simulink model "IBSMC_f"  (R2016b)
settings: Solver=VariableStepAuto  StartTime=0.0  StopTime=0.1  RelTol=1e-3
values from neighbouring files (symbols this model uses):
  a1 = 0.5*eye(3)    [cons2.m]
  a2 = 0.5*eye(3)    [cons2.m]
  j = diag([2.35e-3 2.35e-3 5.26e-2])    [cons2.m]
  k1 = 0.5*eye(3)    [cons2.m]
  k2 = 10*eye(3)    [cons2.m]
undefined symbols (not defined in the file or in its folder): q1, q2
libraries: aerolibutil x1
settings Model: Creator=Ali  LastModifiedBy=Ali

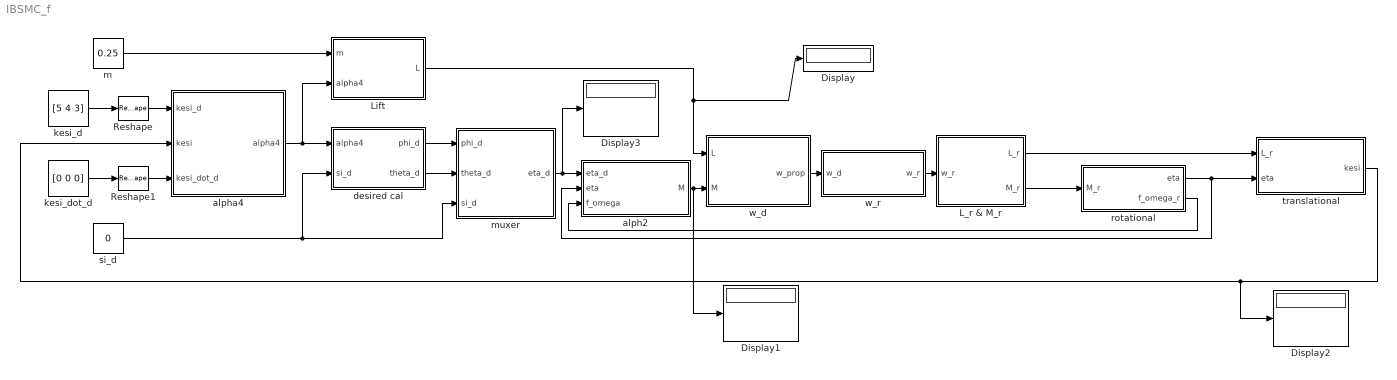
== system IBSMC_f ==
  Display{,1..3} (4 alike) : Display
  L_r & M_r : MATLAB Function  TreatAsAtomicUnit=on
  Lift : MATLAB Function  TreatAsAtomicUnit=on
  Reshape : Reshape  OutputDimensionality=Column vector (2-D)
  Reshape1 : Reshape  OutputDimensionality=Column vector (2-D)
  alph2 : Subsystem
  alpha4 : Subsystem
  desired cal : MATLAB Function  TreatAsAtomicUnit=on
  kesi_d : Constant  Value=[5 4 3]
  kesi_dot_d : Constant  Value=[0 0 0]
  m : Constant  Value=0.25
  muxer : MATLAB Function  TreatAsAtomicUnit=on
  rotational : Subsystem
  si_d : Constant  Value=0
  translational : Subsystem
  w_d : MATLAB Function  TreatAsAtomicUnit=on
  w_r : Subsystem
  wires:
  si_d/1 -> muxer/3(si_d), desired cal/2(si_d)
  desired cal/1(phi_d) -> muxer/1(phi_d)
  desired cal/2(theta_d) -> muxer/2(theta_d)
  muxer/1(eta_d) -> Display3/1, alph2/1(eta_d)
  alpha4/1(alpha4) -> desired cal/1(alpha4), Lift/2(alpha4)
  m/1 -> Lift/1(m)
  alph2/1(M) -> Display1/1, w_d/2(M)
  Lift/1(L) -> Display/1, w_d/1(L)
  w_d/1(w_prop) -> w_r/1(w_d)
  w_r/1(w_r) -> L_r & M_r/1(w_r)
  L_r & M_r/2(M_r) -> rotational/1(M_r)
  rotational/2(f_omega_r) -> alph2/3(f_omega)
  rotational/1(eta) -> alph2/2(eta), translational/2(eta)
  L_r & M_r/1(L_r) -> translational/1(L_r)
  translational/1(kesi) -> alpha4/2(kesi), Display2/1
  Reshape/1 -> alpha4/1(kesi_d)
  kesi_d/1 -> Reshape/1
  Reshape1/1 -> alpha4/3(kesi_dot_d)
  kesi_dot_d/1 -> Reshape1/1

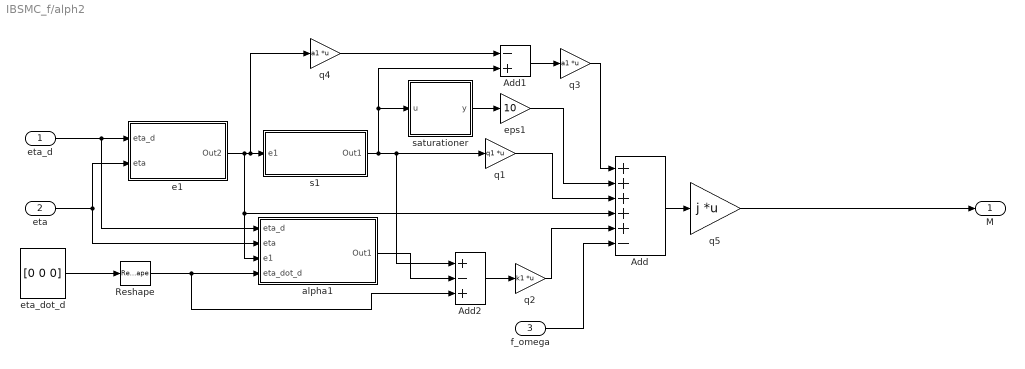
== system IBSMC_f/alph2 ==
  eta_d : Inport
  eta : Inport  Port=2
  f_omega : Inport  Port=3
  Add : Sum  Inputs=+++++-
  Add1 : Sum  Inputs=-+
  Add2 : Sum  Inputs=+-+
  Reshape : Reshape  OutputDimensionality=Column vector (2-D)
  alpha1 : Subsystem
  e1 : Subsystem
  eps1 : Gain  Gain=10
  eta_dot_d : Constant  Value=[0 0 0]
  q1 : Gain  Gain=q1  Multiplication=Matrix(K*u)
  q2 : Gain  Gain=k1  Multiplication=Matrix(K*u)
  q3 : Gain  Gain=a1  Multiplication=Matrix(K*u)
  q4 : Gain  Gain=a1  Multiplication=Matrix(K*u)
  q5 : Gain  Gain=j  Multiplication=Matrix(K*u)
  s1 : Subsystem
  saturationer : MATLAB Function  TreatAsAtomicUnit=on
  M : Outport
  wires:
  eta_d/1 -> alpha1/1(eta_d), e1/1(eta_d)
  e1/1(Out2) -> q4/1, s1/1(e1), alpha1/3(e1), Add/4
  eta_dot_d/1 -> Reshape/1
  saturationer/1(y) -> eps1/1
  s1/1(Out1) -> q1/1, Add2/1, saturationer/1(u), Add1/2
  q5/1 -> M/1
  q1/1 -> Add/3
  eps1/1 -> Add/2
  f_omega/1 -> Add/6
  alpha1/1(Out1) -> Add2/2
  Add2/1 -> q2/1
  q2/1 -> Add/5
  q3/1 -> Add/1
  Add1/1 -> q3/1
  q4/1 -> Add1/1
  eta/1 -> e1/2(eta), alpha1/2(eta)
  Add/1 -> q5/1
  Reshape/1 -> Add2/3, alpha1/4(eta_dot_d)

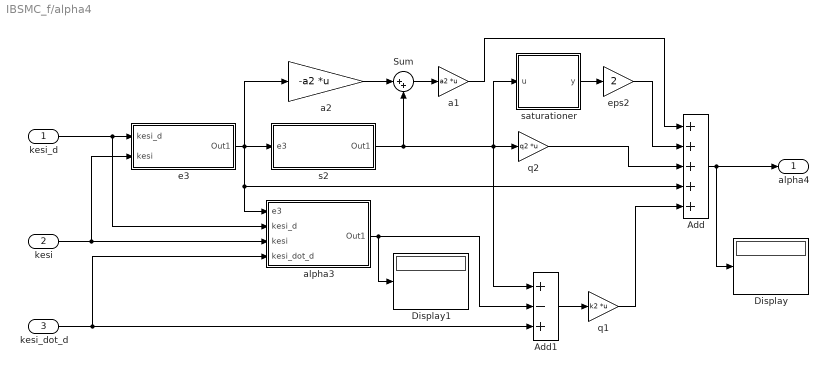
== system IBSMC_f/alpha4 ==
  kesi_d : Inport
  kesi : Inport  Port=2
  kesi_dot_d : Inport  Port=3
  Add : Sum  Inputs=+++++
  Add1 : Sum  Inputs=+-+
  Display : Display
  Display1 : Display
  Sum : Sum  Inputs=|++
  a1 : Gain  Gain=a2  Multiplication=Matrix(K*u)
  a2 : Gain  Gain=-a2  Multiplication=Matrix(K*u)
  alpha3 : Subsystem
  e3 : Subsystem
  eps2 : Gain  Gain=2
  q1 : Gain  Gain=k2  Multiplication=Matrix(K*u)
  q2 : Gain  Gain=q2  Multiplication=Matrix(K*u)
  s2 : Subsystem
  saturationer : MATLAB Function  TreatAsAtomicUnit=on
  alpha4 : Outport
  wires:
  saturationer/1(y) -> eps2/1
  q2/1 -> Add/3
  alpha3/1(Out1) -> Add1/2, Display1/1
  kesi/1 -> e3/2(kesi), alpha3/3(kesi)
  s2/1(Out1) -> q2/1, saturationer/1(u), Add1/1, Sum/2
  e3/1(Out1) -> s2/1(e3), alpha3/1(e3), Add/4, a2/1
  kesi_dot_d/1 -> alpha3/4(kesi_dot_d), Add1/3
  kesi_d/1 -> e3/1(kesi_d), alpha3/2(kesi_d)
  a2/1 -> Sum/1
  Sum/1 -> a1/1
  Add/1 -> alpha4/1, Display/1
  a1/1 -> Add/1
  Add1/1 -> q1/1
  q1/1 -> Add/5
  eps2/1 -> Add/2

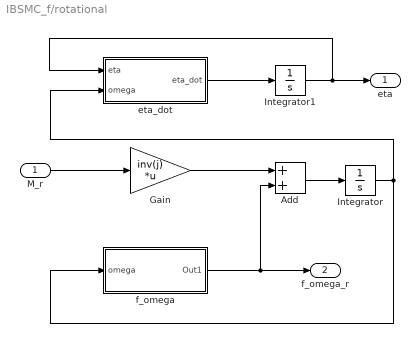
== system IBSMC_f/rotational ==
  M_r : Inport
  Add : Sum
  Gain : Gain  Gain=inv(j)  Multiplication=Matrix(K*u)
  Integrator : Integrator
  Integrator1 : Integrator
  eta_dot : Subsystem
  f_omega : Subsystem
  eta : Outport
  f_omega_r : Outport  Port=2
  wires:
  M_r/1 -> Gain/1
  Gain/1 -> Add/1
  Add/1 -> Integrator/1
  f_omega/1(Out1) -> Add/2, f_omega_r/1
  Integrator/1 -> f_omega/1(omega), eta_dot/2(omega)
  eta_dot/1(eta_dot) -> Integrator1/1
  Integrator1/1 -> eta/1, eta_dot/1(eta)

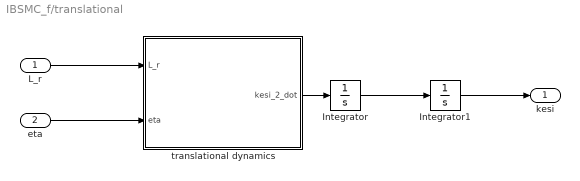
== system IBSMC_f/translational ==
  L_r : Inport
  eta : Inport  Port=2
  Integrator : Integrator
  Integrator1 : Integrator
  translational dynamics : MATLAB Function  TreatAsAtomicUnit=on
  kesi : Outport
  wires:
  L_r/1 -> translational dynamics/1(L_r)
  eta/1 -> translational dynamics/2(eta)
  Integrator/1 -> Integrator1/1
  translational dynamics/1(kesi_2_dot) -> Integrator/1
  Integrator1/1 -> kesi/1

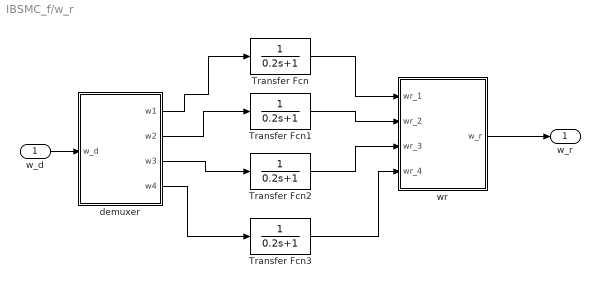
== system IBSMC_f/w_r ==
  w_d : Inport
  Transfer Fcn{,1..3} (4 alike) : TransferFcn  Denominator=[0.2 1]
  demuxer : MATLAB Function  TreatAsAtomicUnit=on
  wr : MATLAB Function  TreatAsAtomicUnit=on
  w_r : Outport
  wires:
  w_d/1 -> demuxer/1(w_d)
  demuxer/1(w1) -> Transfer Fcn/1
  demuxer/2(w2) -> Transfer Fcn1/1
  demuxer/3(w3) -> Transfer Fcn2/1
  demuxer/4(w4) -> Transfer Fcn3/1
  Transfer Fcn/1 -> wr/1(wr_1)
  Transfer Fcn1/1 -> wr/2(wr_2)
  Transfer Fcn2/1 -> wr/3(wr_3)
  Transfer Fcn3/1 -> wr/4(wr_4)
  wr/1(w_r) -> w_r/1

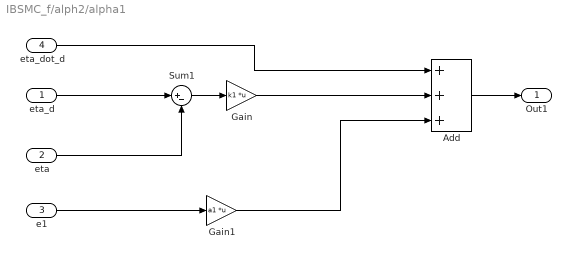
== system IBSMC_f/alph2/alpha1 ==
  eta_d : Inport
  eta : Inport  Port=2
  e1 : Inport  Port=3
  eta_dot_d : Inport  Port=4
  Add : Sum  Inputs=+++
  Gain : Gain  Gain=k1  Multiplication=Matrix(K*u)
  Gain1 : Gain  Gain=a1  Multiplication=Matrix(K*u)
  Sum1 : Sum  Inputs=|+-
  Out1 : Outport
  wires:
  Add/1 -> Out1/1
  Sum1/1 -> Gain/1
  eta/1 -> Sum1/2
  eta_d/1 -> Sum1/1
  Gain/1 -> Add/2
  eta_dot_d/1 -> Add/1
  e1/1 -> Gain1/1
  Gain1/1 -> Add/3

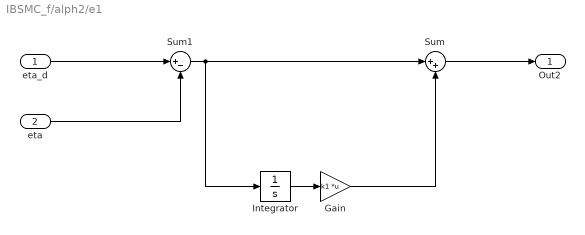
== system IBSMC_f/alph2/e1 ==
  eta_d : Inport
  eta : Inport  Port=2
  Gain : Gain  Gain=k1  Multiplication=Matrix(K*u)
  Integrator : Integrator
  Sum : Sum  Inputs=|++
  Sum1 : Sum  Inputs=|+-
  Out2 : Outport
  wires:
  eta_d/1 -> Sum1/1
  eta/1 -> Sum1/2
  Sum1/1 -> Integrator/1, Sum/1
  Sum/1 -> Out2/1
  Gain/1 -> Sum/2
  Integrator/1 -> Gain/1

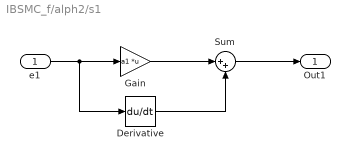
== system IBSMC_f/alph2/s1 ==
  e1 : Inport
  Derivative : Derivative
  Gain : Gain  Gain=a1  Multiplication=Matrix(K*u)
  Sum : Sum  Inputs=|++
  Out1 : Outport
  wires:
  Sum/1 -> Out1/1
  e1/1 -> Derivative/1, Gain/1
  Gain/1 -> Sum/1
  Derivative/1 -> Sum/2

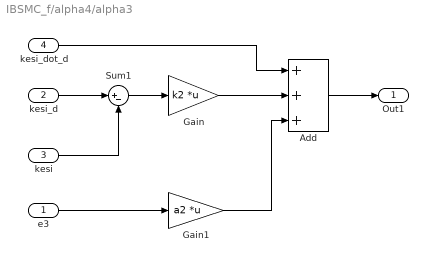
== system IBSMC_f/alpha4/alpha3 ==
  e3 : Inport
  kesi_d : Inport  Port=2
  kesi : Inport  Port=3
  kesi_dot_d : Inport  Port=4
  Add : Sum  Inputs=+++
  Gain : Gain  Gain=k2  Multiplication=Matrix(K*u)
  Gain1 : Gain  Gain=a2  Multiplication=Matrix(K*u)
  Sum1 : Sum  Inputs=|+-
  Out1 : Outport
  wires:
  Add/1 -> Out1/1
  Sum1/1 -> Gain/1
  kesi/1 -> Sum1/2
  kesi_d/1 -> Sum1/1
  Gain/1 -> Add/2
  kesi_dot_d/1 -> Add/1
  e3/1 -> Gain1/1
  Gain1/1 -> Add/3

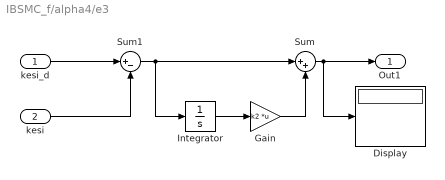
== system IBSMC_f/alpha4/e3 ==
  kesi_d : Inport
  kesi : Inport  Port=2
  Display : Display
  Gain : Gain  Gain=k2  Multiplication=Matrix(K*u)
  Integrator : Integrator
  Sum : Sum  Inputs=|++
  Sum1 : Sum  Inputs=|+-
  Out1 : Outport
  wires:
  kesi_d/1 -> Sum1/1
  kesi/1 -> Sum1/2
  Sum1/1 -> Integrator/1, Sum/1
  Integrator/1 -> Gain/1
  Gain/1 -> Sum/2
  Sum/1 -> Out1/1, Display/1

== system IBSMC_f/alpha4/s2 ==
  e3 : Inport
  Derivative : Derivative
  Gain : Gain  Gain=a2  Multiplication=Matrix(K*u)
  Sum : Sum  Inputs=|++
  Out1 : Outport
  wires:
  Sum/1 -> Out1/1
  e3/1 -> Derivative/1, Gain/1
  Gain/1 -> Sum/1
  Derivative/1 -> Sum/2

== system IBSMC_f/rotational/eta_dot ==
  eta : Inport
  omega : Inport  Port=2
  eta_dot_cal : MATLAB Function  TreatAsAtomicUnit=on
  eta_dot : Outport
  wires:
  eta_dot_cal/1(eta_dot) -> eta_dot/1
  eta/1 -> eta_dot_cal/1(eta)
  omega/1 -> eta_dot_cal/2(omega)

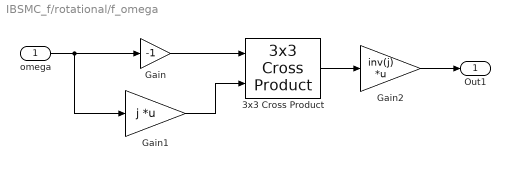
== system IBSMC_f/rotational/f_omega ==
  omega : Inport
  3x3 Cross Product : aerolibutil/3x3 Cross Product
  Gain : Gain  Gain=-1
  Gain1 : Gain  Gain=j  Multiplication=Matrix(K*u)
  Gain2 : Gain  Gain=inv(j)  Multiplication=Matrix(K*u)
  Out1 : Outport
  wires:
  omega/1 -> Gain1/1, Gain/1
  Gain/1 -> 3x3 Cross Product/1
  Gain1/1 -> 3x3 Cross Product/2
  3x3 Cross Product/1 -> Gain2/1
  Gain2/1 -> Out1/1

== matlab function IBSMC_f/desired cal ==
  data: alpha4 input; phi_d output; theta_d output; si_d input
function [phi_d,theta_d] = fcn(alpha4,si_d)
g=9.81;
phi_d=asin((alpha4(1)*sin(si_d)-alpha4(2)*cos(si_d))/sqrt(alpha4(1)^2+alpha4(2)^2+(alpha4(3)+g)^2));
theta_d = atan((alpha4(1)*cos(si_d)+alpha4(2)*sin(si_d))/(alpha4(3)+g));

== matlab function IBSMC_f/Lift ==
  data: m input; alpha4 input; L output
function L = fcn(m,alpha4)
g=9.81;
L = sqrt(m^2*(alpha4(1)^2+alpha4(2)^2+(alpha4(3)+g)^2));

== matlab function IBSMC_f/muxer ==
  data: phi_d input; eta_d output; theta_d input; si_d input
function eta_d = fcn(phi_d,theta_d,si_d)
eta_d = [phi_d;theta_d;si_d];

== matlab function IBSMC_f/w_d ==
  data: L input; w_prop output; M input
function w_prop = fcn(L,M)
b=6.13e-5;d=0.2;kd=2.5e-6;
co=[b b b b;0 -d*b 0 d*b;-d*b 0 d*b 0;kd -kd -kd -kd];
w_prop=sqrt(abs(inv(co)*[L;M]));

== matlab function IBSMC_f/w_r/demuxer ==
  data: w_d input; w1 output; w2 output; w3 output; w4 output
function [w1,w2,w3,w4]= fcn(w_d)
w1=w_d(1);
w2=w_d(2);
w3=w_d(3);
w4=w_d(4);

== matlab function IBSMC_f/w_r/wr ==
  data: wr_1 input; w_r output; wr_2 input; wr_3 input; wr_4 input
function w_r = fcn(wr_1,wr_2,wr_3,wr_4)
w_r =[wr_1;wr_2;wr_3;wr_4];

== matlab function IBSMC_f/L_r & M_r ==
  data: w_r input; L_r output; M_r output
function [L_r,M_r]= fcn(w_r)
b=6.13e-5;d=0.2;kd=2.5e-6;
co=[b b b b;0 -d*b 0 d*b;-d*b 0 d*b 0;kd -kd -kd -kd];
ML=co*w_r.^2;
L_r=ML(1);
M_r=ML(2:4);

== matlab function IBSMC_f/rotational/eta_dot/eta_dot_cal ==
  data: eta input; eta_dot output; omega input
function eta_dot = fcn(eta,omega)
eta_dot=zeros(3,1);
phi=eta(1);
theta=eta(2);
w=[1 sin(phi)*tan(theta) cos(phi)*tan(theta);0 cos(phi) -sin(phi);0 sin(phi)/cos(theta) cos(phi)/cos(theta)];
eta_dot = w*omega;

== matlab function IBSMC_f/translational/translational dynamics ==
  data: L_r input; kesi_2_dot output; eta input
function kesi_2_dot = fcn(L_r,eta)
kesi_2_dot=zeros(3,1);
m=0.25;g=9.81;
r_be=[cos(eta(3))*cos(eta(2)) cos(eta(2))*sin(eta(3)) -sin(eta(2));cos(eta(3))*sin(eta(1))*sin(eta(2))-cos(eta(1))*sin(eta(3)) cos(eta(1))*cos(eta(3))+sin(eta(1))*sin(eta(3))*sin(eta(2)) cos(eta(2))*sin(eta(1));sin(eta(1))*sin(eta(3))+cos(eta(1))*cos(eta(3))*sin(eta(2)) cos(eta(1))*sin(eta(3))*sin(eta(2))-cos(eta(3))*sin(eta(1)) cos(eta(1))*cos(eta(2))];
r_eb=r_be';
kesi_2_dot =r_eb*[0;0;L_r/m]+[0;0;-g];

== matlab function IBSMC_f/alpha4/saturationer ==
  data: u input; y output
function y = fcn(u)
y=min(max(u*0.1,-[1;1;1]),[1;1;1]);

== matlab function IBSMC_f/alph2/saturationer ==
  data: u input; y output
function y = fcn(u)
y=min(max(u*0.1,-[1;1;1]),[1;1;1]);
